simulink model "c00011M_harness"  (R2018a)
settings: Solver=FixedStepAuto  StartTime=0.0  StopTime=300  FixedStep=0.1  RelTol=1e-3
undefined symbols (not defined in the file): A1, hmax, PriorityTank, R1, R2, sigbuilder_block
(part 16 of 73)

== system c00011M_harness/M088/Tank2 ==
  CT2 : Inport
  MR2 : Inport  Port=2
  T2 : Inport  Port=3
  EB2 : Inport  Port=4
  LL1 : Inport  Port=5
  LL3 : Inport  Port=6
  Control : Subsystem
  Logical Operator : Logic  AllPortsSameDT=off  OutDataTypeStr=boolean
  MasterTankControl : Subsystem
  Memory : Memory
  Memory1 : Memory
  Memory2 : Memory
  TankModel : Subsystem
  LL2 : Outport
  wires:
  TankModel/1(LiquidLevel) -> Memory/1, LL2/1
  Control/1(LiquidIn) -> Logical Operator/1
  Control/2(LiquidOut) -> TankModel/2(LiquidOut)
  Memory/1 -> Control/5(LiquidLevel), MasterTankControl/2(LiquidTank2)
  MR2/1 -> Control/3(ManualReference)
  CT2/1 -> Control/2(StartMaintenance), Control/1(ControlType)
  LL3/1 -> Memory2/1
  Memory2/1 -> MasterTankControl/3(LiquidTank3)
  Memory1/1 -> MasterTankControl/1(LiquidTank1)
  EB2/1 -> Control/4(EmergencyButton)
  MasterTankControl/1(AllowTheTankFilling) -> Logical Operator/2
  Logical Operator/1 -> TankModel/1(LiquidIn)
  LL1/1 -> Memory1/1

== system c00011M_harness/M088/Tank3 ==
  CT3 : Inport
  F3 : Inport  Port=2
  E3 : Inport  Port=3
  T3 : Inport  Port=4
  EB3 : Inport  Port=5
  LL1 : Inport  Port=6
  LL2 : Inport  Port=7
  Control : Subsystem
  Logical Operator : Logic  AllPortsSameDT=off  OutDataTypeStr=boolean
  MasterTankControl : Subsystem
  Memory : Memory
  Memory1 : Memory
  Memory2 : Memory
  TankModel : Subsystem
  LL3 : Outport
  wires:
  TankModel/1(LiquidLevel) -> Memory/1, LL3/1
  Control/1(LiquidIn) -> Logical Operator/1
  Control/2(LiquidOut) -> TankModel/2(LiquidOut)
  Memory/1 -> MasterTankControl/3(LiquidTank3), Control/5(LiquidLevel)
  CT3/1 -> Control/1(ControlType)
  F3/1 -> Control/2(Fill)
  E3/1 -> Control/3(Empty)
  LL2/1 -> Memory2/1
  Memory2/1 -> MasterTankControl/2(LiquidTank2)
  Memory1/1 -> MasterTankControl/1(LiquidTank1)
  EB3/1 -> Control/4(EmergencyButton)
  MasterTankControl/1(AllowTheTankFilling) -> Logical Operator/2
  Logical Operator/1 -> TankModel/1(LiquidIn)
  LL1/1 -> Memory1/1

== system c00011M_harness/M089/Tank1 ==
  CT1 : Inport
  MR1 : Inport  Port=2
  T1 : Inport  Port=3
  EB1 : Inport  Port=4
  LL2 : Inport  Port=5
  LL3 : Inport  Port=6
  Control : Subsystem
  Logical Operator : Logic  AllPortsSameDT=off  OutDataTypeStr=boolean
  MasterTankControl : Subsystem
  Memory : Memory
  Memory1 : Memory
  Memory2 : Memory
  TankModel : Subsystem
  LL1 : Outport
  wires:
  TankModel/1(LiquidLevel) -> Memory/1, LL1/1
  Control/1(LiquidIn) -> Logical Operator/1
  Control/2(LiquidOut) -> TankModel/2(LiquidOut)
  Memory/1 -> Control/5(LiquidLevel), MasterTankControl/1(LiquidTank1)
  MR1/1 -> Control/3(ManualReference)
  CT1/1 -> Control/2(StartMaintenance), Control/1(ControlType)
  LL3/1 -> Memory2/1
  Memory2/1 -> MasterTankControl/3(LiquidTank3)
  Memory1/1 -> MasterTankControl/2(LiquidTank2)
  EB1/1 -> Control/4(EmergencyButton)
  MasterTankControl/1(AllowTheTankFilling) -> Logical Operator/2
  Logical Operator/1 -> TankModel/1(LiquidIn)
  LL2/1 -> Memory1/1

== system c00011M_harness/M089/Tank2 ==
  CT2 : Inport
  MR2 : Inport  Port=2
  T2 : Inport  Port=3
  EB2 : Inport  Port=4
  LL1 : Inport  Port=5
  LL3 : Inport  Port=6
  Control : Subsystem
  Logical Operator : Logic  AllPortsSameDT=off  OutDataTypeStr=boolean
  MasterTankControl : Subsystem
  Memory : Memory
  Memory1 : Memory
  Memory2 : Memory
  TankModel : Subsystem
  LL2 : Outport
  wires:
  TankModel/1(LiquidLevel) -> Memory/1, LL2/1
  Control/1(LiquidIn) -> Logical Operator/1
  Control/2(LiquidOut) -> TankModel/2(LiquidOut)
  Memory/1 -> Control/5(LiquidLevel), MasterTankControl/2(LiquidTank2)
  MR2/1 -> Control/3(ManualReference)
  CT2/1 -> Control/2(StartMaintenance), Control/1(ControlType)
  LL3/1 -> Memory2/1
  Memory2/1 -> MasterTankControl/3(LiquidTank3)
  Memory1/1 -> MasterTankControl/1(LiquidTank1)
  EB2/1 -> Control/4(EmergencyButton)
  MasterTankControl/1(AllowTheTankFilling) -> Logical Operator/2
  Logical Operator/1 -> TankModel/1(LiquidIn)
  LL1/1 -> Memory1/1

== system c00011M_harness/M089/Tank3 ==
  CT3 : Inport
  F3 : Inport  Port=2
  E3 : Inport  Port=3
  T3 : Inport  Port=4
  EB3 : Inport  Port=5
  LL1 : Inport  Port=6
  LL2 : Inport  Port=7
  Control : Subsystem
  Logical Operator : Logic  AllPortsSameDT=off  OutDataTypeStr=boolean
  MasterTankControl : Subsystem
  Memory : Memory
  Memory1 : Memory
  Memory2 : Memory
  TankModel : Subsystem
  LL3 : Outport
  wires:
  TankModel/1(LiquidLevel) -> Memory/1, LL3/1
  Control/1(LiquidIn) -> Logical Operator/1
  Control/2(LiquidOut) -> TankModel/2(LiquidOut)
  Memory/1 -> MasterTankControl/3(LiquidTank3), Control/5(LiquidLevel)
  CT3/1 -> Control/1(ControlType)
  F3/1 -> Control/2(Fill)
  E3/1 -> Control/3(Empty)
  LL2/1 -> Memory2/1
  Memory2/1 -> MasterTankControl/2(LiquidTank2)
  Memory1/1 -> MasterTankControl/1(LiquidTank1)
  EB3/1 -> Control/4(EmergencyButton)
  MasterTankControl/1(AllowTheTankFilling) -> Logical Operator/2
  Logical Operator/1 -> TankModel/1(LiquidIn)
  LL1/1 -> Memory1/1

== system c00011M_harness/M090/Tank1 ==
  CT1 : Inport
  MR1 : Inport  Port=2
  T1 : Inport  Port=3
  EB1 : Inport  Port=4
  LL2 : Inport  Port=5
  LL3 : Inport  Port=6
  Control : Subsystem
  Logical Operator : Logic  AllPortsSameDT=off  OutDataTypeStr=boolean
  MasterTankControl : Subsystem
  Memory : Memory
  Memory1 : Memory
  Memory2 : Memory
  TankModel : Subsystem
  LL1 : Outport
  wires:
  TankModel/1(LiquidLevel) -> Memory/1, LL1/1
  Control/1(LiquidIn) -> Logical Operator/1
  Control/2(LiquidOut) -> TankModel/2(LiquidOut)
  Memory/1 -> Control/5(LiquidLevel), MasterTankControl/1(LiquidTank1)
  MR1/1 -> Control/3(ManualReference)
  CT1/1 -> Control/2(StartMaintenance), Control/1(ControlType)
  LL3/1 -> Memory2/1
  Memory2/1 -> MasterTankControl/3(LiquidTank3)
  Memory1/1 -> MasterTankControl/2(LiquidTank2)
  EB1/1 -> Control/4(EmergencyButton)
  MasterTankControl/1(AllowTheTankFilling) -> Logical Operator/2
  Logical Operator/1 -> TankModel/1(LiquidIn)
  LL2/1 -> Memory1/1

== system c00011M_harness/M090/Tank2 ==
  CT2 : Inport
  MR2 : Inport  Port=2
  T2 : Inport  Port=3
  EB2 : Inport  Port=4
  LL1 : Inport  Port=5
  LL3 : Inport  Port=6
  Control : Subsystem
  Logical Operator : Logic  AllPortsSameDT=off  OutDataTypeStr=boolean
  MasterTankControl : Subsystem
  Memory : Memory
  Memory1 : Memory
  Memory2 : Memory
  TankModel : Subsystem
  LL2 : Outport
  wires:
  TankModel/1(LiquidLevel) -> Memory/1, LL2/1
  Control/1(LiquidIn) -> Logical Operator/1
  Control/2(LiquidOut) -> TankModel/2(LiquidOut)
  Memory/1 -> Control/5(LiquidLevel), MasterTankControl/2(LiquidTank2)
  MR2/1 -> Control/3(ManualReference)
  CT2/1 -> Control/2(StartMaintenance), Control/1(ControlType)
  LL3/1 -> Memory2/1
  Memory2/1 -> MasterTankControl/3(LiquidTank3)
  Memory1/1 -> MasterTankControl/1(LiquidTank1)
  EB2/1 -> Control/4(EmergencyButton)
  MasterTankControl/1(AllowTheTankFilling) -> Logical Operator/2
  Logical Operator/1 -> TankModel/1(LiquidIn)
  LL1/1 -> Memory1/1

== system c00011M_harness/M090/Tank3 ==
  CT3 : Inport
  F3 : Inport  Port=2
  E3 : Inport  Port=3
  T3 : Inport  Port=4
  EB3 : Inport  Port=5
  LL1 : Inport  Port=6
  LL2 : Inport  Port=7
  Control : Subsystem
  Logical Operator : Logic  AllPortsSameDT=off  OutDataTypeStr=boolean
  MasterTankControl : Subsystem
  Memory : Memory
  Memory1 : Memory
  Memory2 : Memory
  TankModel : Subsystem
  LL3 : Outport
  wires:
  TankModel/1(LiquidLevel) -> Memory/1, LL3/1
  Control/1(LiquidIn) -> Logical Operator/1
  Control/2(LiquidOut) -> TankModel/2(LiquidOut)
  Memory/1 -> MasterTankControl/3(LiquidTank3), Control/5(LiquidLevel)
  CT3/1 -> Control/1(ControlType)
  F3/1 -> Control/2(Fill)
  E3/1 -> Control/3(Empty)
  LL2/1 -> Memory2/1
  Memory2/1 -> MasterTankControl/2(LiquidTank2)
  Memory1/1 -> MasterTankControl/1(LiquidTank1)
  EB3/1 -> Control/4(EmergencyButton)
  MasterTankControl/1(AllowTheTankFilling) -> Logical Operator/2
  Logical Operator/1 -> TankModel/1(LiquidIn)
  LL1/1 -> Memory1/1

== system c00011M_harness/M091/Tank1 ==
  CT1 : Inport
  MR1 : Inport  Port=2
  T1 : Inport  Port=3
  EB1 : Inport  Port=4
  LL2 : Inport  Port=5
  LL3 : Inport  Port=6
  Control : Subsystem
  Logical Operator : Logic  AllPortsSameDT=off  OutDataTypeStr=boolean
  MasterTankControl : Subsystem
  Memory : Memory
  Memory1 : Memory
  Memory2 : Memory
  TankModel : Subsystem
  LL1 : Outport
  wires:
  TankModel/1(LiquidLevel) -> Memory/1, LL1/1
  Control/1(LiquidIn) -> Logical Operator/1
  Control/2(LiquidOut) -> TankModel/2(LiquidOut)
  Memory/1 -> Control/5(LiquidLevel), MasterTankControl/1(LiquidTank1)
  MR1/1 -> Control/3(ManualReference)
  CT1/1 -> Control/2(StartMaintenance), Control/1(ControlType)
  LL3/1 -> Memory2/1
  Memory2/1 -> MasterTankControl/3(LiquidTank3)
  Memory1/1 -> MasterTankControl/2(LiquidTank2)
  EB1/1 -> Control/4(EmergencyButton)
  MasterTankControl/1(AllowTheTankFilling) -> Logical Operator/2
  Logical Operator/1 -> TankModel/1(LiquidIn)
  LL2/1 -> Memory1/1

== system c00011M_harness/M091/Tank2 ==
  CT2 : Inport
  MR2 : Inport  Port=2
  T2 : Inport  Port=3
  EB2 : Inport  Port=4
  LL1 : Inport  Port=5
  LL3 : Inport  Port=6
  Control : Subsystem
  Logical Operator : Logic  AllPortsSameDT=off  OutDataTypeStr=boolean
  MasterTankControl : Subsystem
  Memory : Memory
  Memory1 : Memory
  Memory2 : Memory
  TankModel : Subsystem
  LL2 : Outport
  wires:
  TankModel/1(LiquidLevel) -> Memory/1, LL2/1
  Control/1(LiquidIn) -> Logical Operator/1
  Control/2(LiquidOut) -> TankModel/2(LiquidOut)
  Memory/1 -> Control/5(LiquidLevel), MasterTankControl/2(LiquidTank2)
  MR2/1 -> Control/3(ManualReference)
  CT2/1 -> Control/2(StartMaintenance), Control/1(ControlType)
  LL3/1 -> Memory2/1
  Memory2/1 -> MasterTankControl/3(LiquidTank3)
  Memory1/1 -> MasterTankControl/1(LiquidTank1)
  EB2/1 -> Control/4(EmergencyButton)
  MasterTankControl/1(AllowTheTankFilling) -> Logical Operator/2
  Logical Operator/1 -> TankModel/1(LiquidIn)
  LL1/1 -> Memory1/1

== system c00011M_harness/M091/Tank3 ==
  CT3 : Inport
  F3 : Inport  Port=2
  E3 : Inport  Port=3
  T3 : Inport  Port=4
  EB3 : Inport  Port=5
  LL1 : Inport  Port=6
  LL2 : Inport  Port=7
  Control : Subsystem
  Logical Operator : Logic  AllPortsSameDT=off  OutDataTypeStr=boolean
  MasterTankControl : Subsystem
  Memory : Memory
  Memory1 : Memory
  Memory2 : Memory
  TankModel : Subsystem
  LL3 : Outport
  wires:
  TankModel/1(LiquidLevel) -> Memory/1, LL3/1
  Control/1(LiquidIn) -> Logical Operator/1
  Control/2(LiquidOut) -> TankModel/2(LiquidOut)
  Memory/1 -> MasterTankControl/3(LiquidTank3), Control/5(LiquidLevel)
  CT3/1 -> Control/1(ControlType)
  F3/1 -> Control/2(Fill)
  E3/1 -> Control/3(Empty)
  LL2/1 -> Memory2/1
  Memory2/1 -> MasterTankControl/2(LiquidTank2)
  Memory1/1 -> MasterTankControl/1(LiquidTank1)
  EB3/1 -> Control/4(EmergencyButton)
  MasterTankControl/1(AllowTheTankFilling) -> Logical Operator/2
  Logical Operator/1 -> TankModel/1(LiquidIn)
  LL1/1 -> Memory1/1

== system c00011M_harness/M092/Tank1 ==
  CT1 : Inport
  MR1 : Inport  Port=2
  T1 : Inport  Port=3
  EB1 : Inport  Port=4
  LL2 : Inport  Port=5
  LL3 : Inport  Port=6
  Control : Subsystem
  Logical Operator : Logic  AllPortsSameDT=off  OutDataTypeStr=boolean
  MasterTankControl : Subsystem
  Memory : Memory
  Memory1 : Memory
  Memory2 : Memory
  TankModel : Subsystem
  LL1 : Outport
  wires:
  TankModel/1(LiquidLevel) -> Memory/1, LL1/1
  Control/1(LiquidIn) -> Logical Operator/1
  Control/2(LiquidOut) -> TankModel/2(LiquidOut)
  Memory/1 -> Control/5(LiquidLevel), MasterTankControl/1(LiquidTank1)
  MR1/1 -> Control/3(ManualReference)
  CT1/1 -> Control/2(StartMaintenance), Control/1(ControlType)
  LL3/1 -> Memory2/1
  Memory2/1 -> MasterTankControl/3(LiquidTank3)
  Memory1/1 -> MasterTankControl/2(LiquidTank2)
  EB1/1 -> Control/4(EmergencyButton)
  MasterTankControl/1(AllowTheTankFilling) -> Logical Operator/2
  Logical Operator/1 -> TankModel/1(LiquidIn)
  LL2/1 -> Memory1/1

== system c00011M_harness/M092/Tank2 ==
  CT2 : Inport
  MR2 : Inport  Port=2
  T2 : Inport  Port=3
  EB2 : Inport  Port=4
  LL1 : Inport  Port=5
  LL3 : Inport  Port=6
  Control : Subsystem
  Logical Operator : Logic  AllPortsSameDT=off  OutDataTypeStr=boolean
  MasterTankControl : Subsystem
  Memory : Memory
  Memory1 : Memory
  Memory2 : Memory
  TankModel : Subsystem
  LL2 : Outport
  wires:
  TankModel/1(LiquidLevel) -> Memory/1, LL2/1
  Control/1(LiquidIn) -> Logical Operator/1
  Control/2(LiquidOut) -> TankModel/2(LiquidOut)
  Memory/1 -> Control/5(LiquidLevel), MasterTankControl/2(LiquidTank2)
  MR2/1 -> Control/3(ManualReference)
  CT2/1 -> Control/2(StartMaintenance), Control/1(ControlType)
  LL3/1 -> Memory2/1
  Memory2/1 -> MasterTankControl/3(LiquidTank3)
  Memory1/1 -> MasterTankControl/1(LiquidTank1)
  EB2/1 -> Control/4(EmergencyButton)
  MasterTankControl/1(AllowTheTankFilling) -> Logical Operator/2
  Logical Operator/1 -> TankModel/1(LiquidIn)
  LL1/1 -> Memory1/1

== system c00011M_harness/M092/Tank3 ==
  CT3 : Inport
  F3 : Inport  Port=2
  E3 : Inport  Port=3
  T3 : Inport  Port=4
  EB3 : Inport  Port=5
  LL1 : Inport  Port=6
  LL2 : Inport  Port=7
  Control : Subsystem
  Logical Operator : Logic  AllPortsSameDT=off  OutDataTypeStr=boolean
  MasterTankControl : Subsystem
  Memory : Memory
  Memory1 : Memory
  Memory2 : Memory
  TankModel : Subsystem
  LL3 : Outport
  wires:
  TankModel/1(LiquidLevel) -> Memory/1, LL3/1
  Control/1(LiquidIn) -> Logical Operator/1
  Control/2(LiquidOut) -> TankModel/2(LiquidOut)
  Memory/1 -> MasterTankControl/3(LiquidTank3), Control/5(LiquidLevel)
  CT3/1 -> Control/1(ControlType)
  F3/1 -> Control/2(Fill)
  E3/1 -> Control/3(Empty)
  LL2/1 -> Memory2/1
  Memory2/1 -> MasterTankControl/2(LiquidTank2)
  Memory1/1 -> MasterTankControl/1(LiquidTank1)
  EB3/1 -> Control/4(EmergencyButton)
  MasterTankControl/1(AllowTheTankFilling) -> Logical Operator/2
  Logical Operator/1 -> TankModel/1(LiquidIn)
  LL1/1 -> Memory1/1

== system c00011M_harness/M093/Tank1 ==
  CT1 : Inport
  MR1 : Inport  Port=2
  T1 : Inport  Port=3
  EB1 : Inport  Port=4
  LL2 : Inport  Port=5
  LL3 : Inport  Port=6
  Control : Subsystem
  Logical Operator : Logic  AllPortsSameDT=off  OutDataTypeStr=boolean
  MasterTankControl : Subsystem
  Memory : Memory
  Memory1 : Memory
  Memory2 : Memory
  TankModel : Subsystem
  LL1 : Outport
  wires:
  TankModel/1(LiquidLevel) -> Memory/1, LL1/1
  Control/1(LiquidIn) -> Logical Operator/1
  Control/2(LiquidOut) -> TankModel/2(LiquidOut)
  Memory/1 -> Control/5(LiquidLevel), MasterTankControl/1(LiquidTank1)
  MR1/1 -> Control/3(ManualReference)
  CT1/1 -> Control/2(StartMaintenance), Control/1(ControlType)
  LL3/1 -> Memory2/1
  Memory2/1 -> MasterTankControl/3(LiquidTank3)
  Memory1/1 -> MasterTankControl/2(LiquidTank2)
  EB1/1 -> Control/4(EmergencyButton)
  MasterTankControl/1(AllowTheTankFilling) -> Logical Operator/2
  Logical Operator/1 -> TankModel/1(LiquidIn)
  LL2/1 -> Memory1/1

== system c00011M_harness/M093/Tank2 ==
  CT2 : Inport
  MR2 : Inport  Port=2
  T2 : Inport  Port=3
  EB2 : Inport  Port=4
  LL1 : Inport  Port=5
  LL3 : Inport  Port=6
  Control : Subsystem
  Logical Operator : Logic  AllPortsSameDT=off  OutDataTypeStr=boolean
  MasterTankControl : Subsystem
  Memory : Memory
  Memory1 : Memory
  Memory2 : Memory
  TankModel : Subsystem
  LL2 : Outport
  wires:
  TankModel/1(LiquidLevel) -> Memory/1, LL2/1
  Control/1(LiquidIn) -> Logical Operator/1
  Control/2(LiquidOut) -> TankModel/2(LiquidOut)
  Memory/1 -> Control/5(LiquidLevel), MasterTankControl/2(LiquidTank2)
  MR2/1 -> Control/3(ManualReference)
  CT2/1 -> Control/2(StartMaintenance), Control/1(ControlType)
  LL3/1 -> Memory2/1
  Memory2/1 -> MasterTankControl/3(LiquidTank3)
  Memory1/1 -> MasterTankControl/1(LiquidTank1)
  EB2/1 -> Control/4(EmergencyButton)
  MasterTankControl/1(AllowTheTankFilling) -> Logical Operator/2
  Logical Operator/1 -> TankModel/1(LiquidIn)
  LL1/1 -> Memory1/1

== system c00011M_harness/M093/Tank3 ==
  CT3 : Inport
  F3 : Inport  Port=2
  E3 : Inport  Port=3
  T3 : Inport  Port=4
  EB3 : Inport  Port=5
  LL1 : Inport  Port=6
  LL2 : Inport  Port=7
  Control : Subsystem
  Logical Operator : Logic  AllPortsSameDT=off  OutDataTypeStr=boolean
  MasterTankControl : Subsystem
  Memory : Memory
  Memory1 : Memory
  Memory2 : Memory
  TankModel : Subsystem
  LL3 : Outport
  wires:
  TankModel/1(LiquidLevel) -> Memory/1, LL3/1
  Control/1(LiquidIn) -> Logical Operator/1
  Control/2(LiquidOut) -> TankModel/2(LiquidOut)
  Memory/1 -> MasterTankControl/3(LiquidTank3), Control/5(LiquidLevel)
  CT3/1 -> Control/1(ControlType)
  F3/1 -> Control/2(Fill)
  E3/1 -> Control/3(Empty)
  LL2/1 -> Memory2/1
  Memory2/1 -> MasterTankControl/2(LiquidTank2)
  Memory1/1 -> MasterTankControl/1(LiquidTank1)
  EB3/1 -> Control/4(EmergencyButton)
  MasterTankControl/1(AllowTheTankFilling) -> Logical Operator/2
  Logical Operator/1 -> TankModel/1(LiquidIn)
  LL1/1 -> Memory1/1

== system c00011M_harness/M094/Tank1 ==
  CT1 : Inport
  MR1 : Inport  Port=2
  T1 : Inport  Port=3
  EB1 : Inport  Port=4
  LL2 : Inport  Port=5
  LL3 : Inport  Port=6
  Control : Subsystem
  Logical Operator : Logic  AllPortsSameDT=off  OutDataTypeStr=boolean
  MasterTankControl : Subsystem
  Memory : Memory
  Memory1 : Memory
  Memory2 : Memory
  TankModel : Subsystem
  LL1 : Outport
  wires:
  TankModel/1(LiquidLevel) -> Memory/1, LL1/1
  Control/1(LiquidIn) -> Logical Operator/1
  Control/2(LiquidOut) -> TankModel/2(LiquidOut)
  Memory/1 -> Control/5(LiquidLevel), MasterTankControl/1(LiquidTank1)
  MR1/1 -> Control/3(ManualReference)
  CT1/1 -> Control/2(StartMaintenance), Control/1(ControlType)
  LL3/1 -> Memory2/1
  Memory2/1 -> MasterTankControl/3(LiquidTank3)
  Memory1/1 -> MasterTankControl/2(LiquidTank2)
  EB1/1 -> Control/4(EmergencyButton)
  MasterTankControl/1(AllowTheTankFilling) -> Logical Operator/2
  Logical Operator/1 -> TankModel/1(LiquidIn)
  LL2/1 -> Memory1/1

== system c00011M_harness/M094/Tank2 ==
  CT2 : Inport
  MR2 : Inport  Port=2
  T2 : Inport  Port=3
  EB2 : Inport  Port=4
  LL1 : Inport  Port=5
  LL3 : Inport  Port=6
  Control : Subsystem
  Logical Operator : Logic  AllPortsSameDT=off  OutDataTypeStr=boolean
  MasterTankControl : Subsystem
  Memory : Memory
  Memory1 : Memory
  Memory2 : Memory
  TankModel : Subsystem
  LL2 : Outport
  wires:
  TankModel/1(LiquidLevel) -> Memory/1, LL2/1
  Control/1(LiquidIn) -> Logical Operator/1
  Control/2(LiquidOut) -> TankModel/2(LiquidOut)
  Memory/1 -> Control/5(LiquidLevel), MasterTankControl/2(LiquidTank2)
  MR2/1 -> Control/3(ManualReference)
  CT2/1 -> Control/2(StartMaintenance), Control/1(ControlType)
  LL3/1 -> Memory2/1
  Memory2/1 -> MasterTankControl/3(LiquidTank3)
  Memory1/1 -> MasterTankControl/1(LiquidTank1)
  EB2/1 -> Control/4(EmergencyButton)
  MasterTankControl/1(AllowTheTankFilling) -> Logical Operator/2
  Logical Operator/1 -> TankModel/1(LiquidIn)
  LL1/1 -> Memory1/1

== system c00011M_harness/M094/Tank3 ==
  CT3 : Inport
  F3 : Inport  Port=2
  E3 : Inport  Port=3
  T3 : Inport  Port=4
  EB3 : Inport  Port=5
  LL1 : Inport  Port=6
  LL2 : Inport  Port=7
  Control : Subsystem
  Logical Operator : Logic  AllPortsSameDT=off  OutDataTypeStr=boolean
  MasterTankControl : Subsystem
  Memory : Memory
  Memory1 : Memory
  Memory2 : Memory
  TankModel : Subsystem
  LL3 : Outport
  wires:
  TankModel/1(LiquidLevel) -> Memory/1, LL3/1
  Control/1(LiquidIn) -> Logical Operator/1
  Control/2(LiquidOut) -> TankModel/2(LiquidOut)
  Memory/1 -> MasterTankControl/3(LiquidTank3), Control/5(LiquidLevel)
  CT3/1 -> Control/1(ControlType)
  F3/1 -> Control/2(Fill)
  E3/1 -> Control/3(Empty)
  LL2/1 -> Memory2/1
  Memory2/1 -> MasterTankControl/2(LiquidTank2)
  Memory1/1 -> MasterTankControl/1(LiquidTank1)
  EB3/1 -> Control/4(EmergencyButton)
  MasterTankControl/1(AllowTheTankFilling) -> Logical Operator/2
  Logical Operator/1 -> TankModel/1(LiquidIn)
  LL1/1 -> Memory1/1

== system c00011M_harness/M095/Tank1 ==
  CT1 : Inport
  MR1 : Inport  Port=2
  T1 : Inport  Port=3
  EB1 : Inport  Port=4
  LL2 : Inport  Port=5
  LL3 : Inport  Port=6
  Control : Subsystem
  Logical Operator : Logic  AllPortsSameDT=off  OutDataTypeStr=boolean
  MasterTankControl : Subsystem
  Memory : Memory
  Memory1 : Memory
  Memory2 : Memory
  TankModel : Subsystem
  LL1 : Outport
  wires:
  TankModel/1(LiquidLevel) -> Memory/1, LL1/1
  Control/1(LiquidIn) -> Logical Operator/1
  Control/2(LiquidOut) -> TankModel/2(LiquidOut)
  Memory/1 -> Control/5(LiquidLevel), MasterTankControl/1(LiquidTank1)
  MR1/1 -> Control/3(ManualReference)
  CT1/1 -> Control/2(StartMaintenance), Control/1(ControlType)
  LL3/1 -> Memory2/1
  Memory2/1 -> MasterTankControl/3(LiquidTank3)
  Memory1/1 -> MasterTankControl/2(LiquidTank2)
  EB1/1 -> Control/4(EmergencyButton)
  MasterTankControl/1(AllowTheTankFilling) -> Logical Operator/2
  Logical Operator/1 -> TankModel/1(LiquidIn)
  LL2/1 -> Memory1/1

== system c00011M_harness/M095/Tank2 ==
  CT2 : Inport
  MR2 : Inport  Port=2
  T2 : Inport  Port=3
  EB2 : Inport  Port=4
  LL1 : Inport  Port=5
  LL3 : Inport  Port=6
  Control : Subsystem
  Logical Operator : Logic  AllPortsSameDT=off  OutDataTypeStr=boolean
  MasterTankControl : Subsystem
  Memory : Memory
  Memory1 : Memory
  Memory2 : Memory
  TankModel : Subsystem
  LL2 : Outport
  wires:
  TankModel/1(LiquidLevel) -> Memory/1, LL2/1
  Control/1(LiquidIn) -> Logical Operator/1
  Control/2(LiquidOut) -> TankModel/2(LiquidOut)
  Memory/1 -> Control/5(LiquidLevel), MasterTankControl/2(LiquidTank2)
  MR2/1 -> Control/3(ManualReference)
  CT2/1 -> Control/2(StartMaintenance), Control/1(ControlType)
  LL3/1 -> Memory2/1
  Memory2/1 -> MasterTankControl/3(LiquidTank3)
  Memory1/1 -> MasterTankControl/1(LiquidTank1)
  EB2/1 -> Control/4(EmergencyButton)
  MasterTankControl/1(AllowTheTankFilling) -> Logical Operator/2
  Logical Operator/1 -> TankModel/1(LiquidIn)
  LL1/1 -> Memory1/1

== system c00011M_harness/M095/Tank3 ==
  CT3 : Inport
  F3 : Inport  Port=2
  E3 : Inport  Port=3
  T3 : Inport  Port=4
  EB3 : Inport  Port=5
  LL1 : Inport  Port=6
  LL2 : Inport  Port=7
  Control : Subsystem
  Logical Operator : Logic  AllPortsSameDT=off  OutDataTypeStr=boolean
  MasterTankControl : Subsystem
  Memory : Memory
  Memory1 : Memory
  Memory2 : Memory
  TankModel : Subsystem
  LL3 : Outport
  wires:
  TankModel/1(LiquidLevel) -> Memory/1, LL3/1
  Control/1(LiquidIn) -> Logical Operator/1
  Control/2(LiquidOut) -> TankModel/2(LiquidOut)
  Memory/1 -> MasterTankControl/3(LiquidTank3), Control/5(LiquidLevel)
  CT3/1 -> Control/1(ControlType)
  F3/1 -> Control/2(Fill)
  E3/1 -> Control/3(Empty)
  LL2/1 -> Memory2/1
  Memory2/1 -> MasterTankControl/2(LiquidTank2)
  Memory1/1 -> MasterTankControl/1(LiquidTank1)
  EB3/1 -> Control/4(EmergencyButton)
  MasterTankControl/1(AllowTheTankFilling) -> Logical Operator/2
  Logical Operator/1 -> TankModel/1(LiquidIn)
  LL1/1 -> Memory1/1

== system c00011M_harness/M096/Tank1 ==
  CT1 : Inport
  MR1 : Inport  Port=2
  T1 : Inport  Port=3
  EB1 : Inport  Port=4
  LL2 : Inport  Port=5
  LL3 : Inport  Port=6
  Control : Subsystem
  Logical Operator : Logic  AllPortsSameDT=off  OutDataTypeStr=boolean
  MasterTankControl : Subsystem
  Memory : Memory
  Memory1 : Memory
  Memory2 : Memory
  TankModel : Subsystem
  LL1 : Outport
  wires:
  TankModel/1(LiquidLevel) -> Memory/1, LL1/1
  Control/1(LiquidIn) -> Logical Operator/1
  Control/2(LiquidOut) -> TankModel/2(LiquidOut)
  Memory/1 -> Control/5(LiquidLevel), MasterTankControl/1(LiquidTank1)
  MR1/1 -> Control/3(ManualReference)
  CT1/1 -> Control/2(StartMaintenance), Control/1(ControlType)
  LL3/1 -> Memory2/1
  Memory2/1 -> MasterTankControl/3(LiquidTank3)
  Memory1/1 -> MasterTankControl/2(LiquidTank2)
  EB1/1 -> Control/4(EmergencyButton)
  MasterTankControl/1(AllowTheTankFilling) -> Logical Operator/2
  Logical Operator/1 -> TankModel/1(LiquidIn)
  LL2/1 -> Memory1/1

== system c00011M_harness/M096/Tank2 ==
  CT2 : Inport
  MR2 : Inport  Port=2
  T2 : Inport  Port=3
  EB2 : Inport  Port=4
  LL1 : Inport  Port=5
  LL3 : Inport  Port=6
  Control : Subsystem
  Logical Operator : Logic  AllPortsSameDT=off  OutDataTypeStr=boolean
  MasterTankControl : Subsystem
  Memory : Memory
  Memory1 : Memory
  Memory2 : Memory
  TankModel : Subsystem
  LL2 : Outport
  wires:
  TankModel/1(LiquidLevel) -> Memory/1, LL2/1
  Control/1(LiquidIn) -> Logical Operator/1
  Control/2(LiquidOut) -> TankModel/2(LiquidOut)
  Memory/1 -> Control/5(LiquidLevel), MasterTankControl/2(LiquidTank2)
  MR2/1 -> Control/3(ManualReference)
  CT2/1 -> Control/2(StartMaintenance), Control/1(ControlType)
  LL3/1 -> Memory2/1
  Memory2/1 -> MasterTankControl/3(LiquidTank3)
  Memory1/1 -> MasterTankControl/1(LiquidTank1)
  EB2/1 -> Control/4(EmergencyButton)
  MasterTankControl/1(AllowTheTankFilling) -> Logical Operator/2
  Logical Operator/1 -> TankModel/1(LiquidIn)
  LL1/1 -> Memory1/1

== system c00011M_harness/M096/Tank3 ==
  CT3 : Inport
  F3 : Inport  Port=2
  E3 : Inport  Port=3
  T3 : Inport  Port=4
  EB3 : Inport  Port=5
  LL1 : Inport  Port=6
  LL2 : Inport  Port=7
  Control : Subsystem
  Logical Operator : Logic  AllPortsSameDT=off  OutDataTypeStr=boolean
  MasterTankControl : Subsystem
  Memory : Memory
  Memory1 : Memory
  Memory2 : Memory
  TankModel : Subsystem
  LL3 : Outport
  wires:
  TankModel/1(LiquidLevel) -> Memory/1, LL3/1
  Control/1(LiquidIn) -> Logical Operator/1
  Control/2(LiquidOut) -> TankModel/2(LiquidOut)
  Memory/1 -> MasterTankControl/3(LiquidTank3), Control/5(LiquidLevel)
  CT3/1 -> Control/1(ControlType)
  F3/1 -> Control/2(Fill)
  E3/1 -> Control/3(Empty)
  LL2/1 -> Memory2/1
  Memory2/1 -> MasterTankControl/2(LiquidTank2)
  Memory1/1 -> MasterTankControl/1(LiquidTank1)
  EB3/1 -> Control/4(EmergencyButton)
  MasterTankControl/1(AllowTheTankFilling) -> Logical Operator/2
  Logical Operator/1 -> TankModel/1(LiquidIn)
  LL1/1 -> Memory1/1

== system c00011M_harness/M097/Tank1 ==
  CT1 : Inport
  MR1 : Inport  Port=2
  T1 : Inport  Port=3
  EB1 : Inport  Port=4
  LL2 : Inport  Port=5
  LL3 : Inport  Port=6
  Control : Subsystem
  Logical Operator : Logic  AllPortsSameDT=off  OutDataTypeStr=boolean
  MasterTankControl : Subsystem
  Memory : Memory
  Memory1 : Memory
  Memory2 : Memory
  TankModel : Subsystem
  LL1 : Outport
  wires:
  TankModel/1(LiquidLevel) -> Memory/1, LL1/1
  Control/1(LiquidIn) -> Logical Operator/1
  Control/2(LiquidOut) -> TankModel/2(LiquidOut)
  Memory/1 -> Control/5(LiquidLevel), MasterTankControl/1(LiquidTank1)
  MR1/1 -> Control/3(ManualReference)
  CT1/1 -> Control/2(StartMaintenance), Control/1(ControlType)
  LL3/1 -> Memory2/1
  Memory2/1 -> MasterTankControl/3(LiquidTank3)
  Memory1/1 -> MasterTankControl/2(LiquidTank2)
  EB1/1 -> Control/4(EmergencyButton)
  MasterTankControl/1(AllowTheTankFilling) -> Logical Operator/2
  Logical Operator/1 -> TankModel/1(LiquidIn)
  LL2/1 -> Memory1/1

== system c00011M_harness/M097/Tank2 ==
  CT2 : Inport
  MR2 : Inport  Port=2
  T2 : Inport  Port=3
  EB2 : Inport  Port=4
  LL1 : Inport  Port=5
  LL3 : Inport  Port=6
  Control : Subsystem
  Logical Operator : Logic  AllPortsSameDT=off  OutDataTypeStr=boolean
  MasterTankControl : Subsystem
  Memory : Memory
  Memory1 : Memory
  Memory2 : Memory
  TankModel : Subsystem
  LL2 : Outport
  wires:
  TankModel/1(LiquidLevel) -> Memory/1, LL2/1
  Control/1(LiquidIn) -> Logical Operator/1
  Control/2(LiquidOut) -> TankModel/2(LiquidOut)
  Memory/1 -> Control/5(LiquidLevel), MasterTankControl/2(LiquidTank2)
  MR2/1 -> Control/3(ManualReference)
  CT2/1 -> Control/2(StartMaintenance), Control/1(ControlType)
  LL3/1 -> Memory2/1
  Memory2/1 -> MasterTankControl/3(LiquidTank3)
  Memory1/1 -> MasterTankControl/1(LiquidTank1)
  EB2/1 -> Control/4(EmergencyButton)
  MasterTankControl/1(AllowTheTankFilling) -> Logical Operator/2
  Logical Operator/1 -> TankModel/1(LiquidIn)
  LL1/1 -> Memory1/1

== system c00011M_harness/M097/Tank3 ==
  CT3 : Inport
  F3 : Inport  Port=2
  E3 : Inport  Port=3
  T3 : Inport  Port=4
  EB3 : Inport  Port=5
  LL1 : Inport  Port=6
  LL2 : Inport  Port=7
  Control : Subsystem
  Logical Operator : Logic  AllPortsSameDT=off  OutDataTypeStr=boolean
  MasterTankControl : Subsystem
  Memory : Memory
  Memory1 : Memory
  Memory2 : Memory
  TankModel : Subsystem
  LL3 : Outport
  wires:
  TankModel/1(LiquidLevel) -> Memory/1, LL3/1
  Control/1(LiquidIn) -> Logical Operator/1
  Control/2(LiquidOut) -> TankModel/2(LiquidOut)
  Memory/1 -> MasterTankControl/3(LiquidTank3), Control/5(LiquidLevel)
  CT3/1 -> Control/1(ControlType)
  F3/1 -> Control/2(Fill)
  E3/1 -> Control/3(Empty)
  LL2/1 -> Memory2/1
  Memory2/1 -> MasterTankControl/2(LiquidTank2)
  Memory1/1 -> MasterTankControl/1(LiquidTank1)
  EB3/1 -> Control/4(EmergencyButton)
  MasterTankControl/1(AllowTheTankFilling) -> Logical Operator/2
  Logical Operator/1 -> TankModel/1(LiquidIn)
  LL1/1 -> Memory1/1

== system c00011M_harness/M098/Tank1 ==
  CT1 : Inport
  MR1 : Inport  Port=2
  T1 : Inport  Port=3
  EB1 : Inport  Port=4
  LL2 : Inport  Port=5
  LL3 : Inport  Port=6
  Control : Subsystem
  Logical Operator : Logic  AllPortsSameDT=off  OutDataTypeStr=boolean
  MasterTankControl : Subsystem
  Memory : Memory
  Memory1 : Memory
  Memory2 : Memory
  TankModel : Subsystem
  LL1 : Outport
  wires:
  TankModel/1(LiquidLevel) -> Memory/1, LL1/1
  Control/1(LiquidIn) -> Logical Operator/1
  Control/2(LiquidOut) -> TankModel/2(LiquidOut)
  Memory/1 -> Control/5(LiquidLevel), MasterTankControl/1(LiquidTank1)
  MR1/1 -> Control/3(ManualReference)
  CT1/1 -> Control/2(StartMaintenance), Control/1(ControlType)
  LL3/1 -> Memory2/1
  Memory2/1 -> MasterTankControl/3(LiquidTank3)
  Memory1/1 -> MasterTankControl/2(LiquidTank2)
  EB1/1 -> Control/4(EmergencyButton)
  MasterTankControl/1(AllowTheTankFilling) -> Logical Operator/2
  Logical Operator/1 -> TankModel/1(LiquidIn)
  LL2/1 -> Memory1/1

== system c00011M_harness/M098/Tank2 ==
  CT2 : Inport
  MR2 : Inport  Port=2
  T2 : Inport  Port=3
  EB2 : Inport  Port=4
  LL1 : Inport  Port=5
  LL3 : Inport  Port=6
  Control : Subsystem
  Logical Operator : Logic  AllPortsSameDT=off  OutDataTypeStr=boolean
  MasterTankControl : Subsystem
  Memory : Memory
  Memory1 : Memory
  Memory2 : Memory
  TankModel : Subsystem
  LL2 : Outport
  wires:
  TankModel/1(LiquidLevel) -> Memory/1, LL2/1
  Control/1(LiquidIn) -> Logical Operator/1
  Control/2(LiquidOut) -> TankModel/2(LiquidOut)
  Memory/1 -> Control/5(LiquidLevel), MasterTankControl/2(LiquidTank2)
  MR2/1 -> Control/3(ManualReference)
  CT2/1 -> Control/2(StartMaintenance), Control/1(ControlType)
  LL3/1 -> Memory2/1
  Memory2/1 -> MasterTankControl/3(LiquidTank3)
  Memory1/1 -> MasterTankControl/1(LiquidTank1)
  EB2/1 -> Control/4(EmergencyButton)
  MasterTankControl/1(AllowTheTankFilling) -> Logical Operator/2
  Logical Operator/1 -> TankModel/1(LiquidIn)
  LL1/1 -> Memory1/1

== system c00011M_harness/M098/Tank3 ==
  CT3 : Inport
  F3 : Inport  Port=2
  E3 : Inport  Port=3
  T3 : Inport  Port=4
  EB3 : Inport  Port=5
  LL1 : Inport  Port=6
  LL2 : Inport  Port=7
  Control : Subsystem
  Logical Operator : Logic  AllPortsSameDT=off  OutDataTypeStr=boolean
  MasterTankControl : Subsystem
  Memory : Memory
  Memory1 : Memory
  Memory2 : Memory
  TankModel : Subsystem
  LL3 : Outport
  wires:
  TankModel/1(LiquidLevel) -> Memory/1, LL3/1
  Control/1(LiquidIn) -> Logical Operator/1
  Control/2(LiquidOut) -> TankModel/2(LiquidOut)
  Memory/1 -> MasterTankControl/3(LiquidTank3), Control/5(LiquidLevel)
  CT3/1 -> Control/1(ControlType)
  F3/1 -> Control/2(Fill)
  E3/1 -> Control/3(Empty)
  LL2/1 -> Memory2/1
  Memory2/1 -> MasterTankControl/2(LiquidTank2)
  Memory1/1 -> MasterTankControl/1(LiquidTank1)
  EB3/1 -> Control/4(EmergencyButton)
  MasterTankControl/1(AllowTheTankFilling) -> Logical Operator/2
  Logical Operator/1 -> TankModel/1(LiquidIn)
  LL1/1 -> Memory1/1

== system c00011M_harness/M099/Tank1 ==
  CT1 : Inport
  MR1 : Inport  Port=2
  T1 : Inport  Port=3
  EB1 : Inport  Port=4
  LL2 : Inport  Port=5
  LL3 : Inport  Port=6
  Control : Subsystem
  Logical Operator : Logic  AllPortsSameDT=off  OutDataTypeStr=boolean
  MasterTankControl : Subsystem
  Memory : Memory
  Memory1 : Memory
  Memory2 : Memory
  TankModel : Subsystem
  LL1 : Outport
  wires:
  TankModel/1(LiquidLevel) -> Memory/1, LL1/1
  Control/1(LiquidIn) -> Logical Operator/1
  Control/2(LiquidOut) -> TankModel/2(LiquidOut)
  Memory/1 -> Control/5(LiquidLevel), MasterTankControl/1(LiquidTank1)
  MR1/1 -> Control/3(ManualReference)
  CT1/1 -> Control/2(StartMaintenance), Control/1(ControlType)
  LL3/1 -> Memory2/1
  Memory2/1 -> MasterTankControl/3(LiquidTank3)
  Memory1/1 -> MasterTankControl/2(LiquidTank2)
  EB1/1 -> Control/4(EmergencyButton)
  MasterTankControl/1(AllowTheTankFilling) -> Logical Operator/2
  Logical Operator/1 -> TankModel/1(LiquidIn)
  LL2/1 -> Memory1/1

== system c00011M_harness/M099/Tank2 ==
  CT2 : Inport
  MR2 : Inport  Port=2
  T2 : Inport  Port=3
  EB2 : Inport  Port=4
  LL1 : Inport  Port=5
  LL3 : Inport  Port=6
  Control : Subsystem
  Logical Operator : Logic  AllPortsSameDT=off  OutDataTypeStr=boolean
  MasterTankControl : Subsystem
  Memory : Memory
  Memory1 : Memory
  Memory2 : Memory
  TankModel : Subsystem
  LL2 : Outport
  wires:
  TankModel/1(LiquidLevel) -> Memory/1, LL2/1
  Control/1(LiquidIn) -> Logical Operator/1
  Control/2(LiquidOut) -> TankModel/2(LiquidOut)
  Memory/1 -> Control/5(LiquidLevel), MasterTankControl/2(LiquidTank2)
  MR2/1 -> Control/3(ManualReference)
  CT2/1 -> Control/2(StartMaintenance), Control/1(ControlType)
  LL3/1 -> Memory2/1
  Memory2/1 -> MasterTankControl/3(LiquidTank3)
  Memory1/1 -> MasterTankControl/1(LiquidTank1)
  EB2/1 -> Control/4(EmergencyButton)
  MasterTankControl/1(AllowTheTankFilling) -> Logical Operator/2
  Logical Operator/1 -> TankModel/1(LiquidIn)
  LL1/1 -> Memory1/1

== system c00011M_harness/M099/Tank3 ==
  CT3 : Inport
  F3 : Inport  Port=2
  E3 : Inport  Port=3
  T3 : Inport  Port=4
  EB3 : Inport  Port=5
  LL1 : Inport  Port=6
  LL2 : Inport  Port=7
  Control : Subsystem
  Logical Operator : Logic  AllPortsSameDT=off  OutDataTypeStr=boolean
  MasterTankControl : Subsystem
  Memory : Memory
  Memory1 : Memory
  Memory2 : Memory
  TankModel : Subsystem
  LL3 : Outport
  wires:
  TankModel/1(LiquidLevel) -> Memory/1, LL3/1
  Control/1(LiquidIn) -> Logical Operator/1
  Control/2(LiquidOut) -> TankModel/2(LiquidOut)
  Memory/1 -> MasterTankControl/3(LiquidTank3), Control/5(LiquidLevel)
  CT3/1 -> Control/1(ControlType)
  F3/1 -> Control/2(Fill)
  E3/1 -> Control/3(Empty)
  LL2/1 -> Memory2/1
  Memory2/1 -> MasterTankControl/2(LiquidTank2)
  Memory1/1 -> MasterTankControl/1(LiquidTank1)
  EB3/1 -> Control/4(EmergencyButton)
  MasterTankControl/1(AllowTheTankFilling) -> Logical Operator/2
  Logical Operator/1 -> TankModel/1(LiquidIn)
  LL1/1 -> Memory1/1

== system c00011M_harness/M100/Tank1 ==
  CT1 : Inport
  MR1 : Inport  Port=2
  T1 : Inport  Port=3
  EB1 : Inport  Port=4
  LL2 : Inport  Port=5
  LL3 : Inport  Port=6
  Control : Subsystem
  Logical Operator : Logic  AllPortsSameDT=off  OutDataTypeStr=boolean
  MasterTankControl : Subsystem
  Memory : Memory
  Memory1 : Memory
  Memory2 : Memory
  TankModel : Subsystem
  LL1 : Outport
  wires:
  TankModel/1(LiquidLevel) -> Memory/1, LL1/1
  Control/1(LiquidIn) -> Logical Operator/1
  Control/2(LiquidOut) -> TankModel/2(LiquidOut)
  Memory/1 -> Control/5(LiquidLevel), MasterTankControl/1(LiquidTank1)
  MR1/1 -> Control/3(ManualReference)
  CT1/1 -> Control/2(StartMaintenance), Control/1(ControlType)
  LL3/1 -> Memory2/1
  Memory2/1 -> MasterTankControl/3(LiquidTank3)
  Memory1/1 -> MasterTankControl/2(LiquidTank2)
  EB1/1 -> Control/4(EmergencyButton)
  MasterTankControl/1(AllowTheTankFilling) -> Logical Operator/2
  Logical Operator/1 -> TankModel/1(LiquidIn)
  LL2/1 -> Memory1/1

== system c00011M_harness/M100/Tank2 ==
  CT2 : Inport
  MR2 : Inport  Port=2
  T2 : Inport  Port=3
  EB2 : Inport  Port=4
  LL1 : Inport  Port=5
  LL3 : Inport  Port=6
  Control : Subsystem
  Logical Operator : Logic  AllPortsSameDT=off  OutDataTypeStr=boolean
  MasterTankControl : Subsystem
  Memory : Memory
  Memory1 : Memory
  Memory2 : Memory
  TankModel : Subsystem
  LL2 : Outport
  wires:
  TankModel/1(LiquidLevel) -> Memory/1, LL2/1
  Control/1(LiquidIn) -> Logical Operator/1
  Control/2(LiquidOut) -> TankModel/2(LiquidOut)
  Memory/1 -> Control/5(LiquidLevel), MasterTankControl/2(LiquidTank2)
  MR2/1 -> Control/3(ManualReference)
  CT2/1 -> Control/2(StartMaintenance), Control/1(ControlType)
  LL3/1 -> Memory2/1
  Memory2/1 -> MasterTankControl/3(LiquidTank3)
  Memory1/1 -> MasterTankControl/1(LiquidTank1)
  EB2/1 -> Control/4(EmergencyButton)
  MasterTankControl/1(AllowTheTankFilling) -> Logical Operator/2
  Logical Operator/1 -> TankModel/1(LiquidIn)
  LL1/1 -> Memory1/1

== system c00011M_harness/M100/Tank3 ==
  CT3 : Inport
  F3 : Inport  Port=2
  E3 : Inport  Port=3
  T3 : Inport  Port=4
  EB3 : Inport  Port=5
  LL1 : Inport  Port=6
  LL2 : Inport  Port=7
  Control : Subsystem
  Logical Operator : Logic  AllPortsSameDT=off  OutDataTypeStr=boolean
  MasterTankControl : Subsystem
  Memory : Memory
  Memory1 : Memory
  Memory2 : Memory
  TankModel : Subsystem
  LL3 : Outport
  wires:
  TankModel/1(LiquidLevel) -> Memory/1, LL3/1
  Control/1(LiquidIn) -> Logical Operator/1
  Control/2(LiquidOut) -> TankModel/2(LiquidOut)
  Memory/1 -> MasterTankControl/3(LiquidTank3), Control/5(LiquidLevel)
  CT3/1 -> Control/1(ControlType)
  F3/1 -> Control/2(Fill)
  E3/1 -> Control/3(Empty)
  LL2/1 -> Memory2/1
  Memory2/1 -> MasterTankControl/2(LiquidTank2)
  Memory1/1 -> MasterTankControl/1(LiquidTank1)
  EB3/1 -> Control/4(EmergencyButton)
  MasterTankControl/1(AllowTheTankFilling) -> Logical Operator/2
  Logical Operator/1 -> TankModel/1(LiquidIn)
  LL1/1 -> Memory1/1

== system c00011M_harness/M101/Tank1 ==
  CT1 : Inport
  MR1 : Inport  Port=2
  T1 : Inport  Port=3
  EB1 : Inport  Port=4
  LL2 : Inport  Port=5
  LL3 : Inport  Port=6
  Control : Subsystem
  Logical Operator : Logic  AllPortsSameDT=off  OutDataTypeStr=boolean
  MasterTankControl : Subsystem
  Memory : Memory
  Memory1 : Memory
  Memory2 : Memory
  TankModel : Subsystem
  LL1 : Outport
  wires:
  TankModel/1(LiquidLevel) -> Memory/1, LL1/1
  Control/1(LiquidIn) -> Logical Operator/1
  Control/2(LiquidOut) -> TankModel/2(LiquidOut)
  Memory/1 -> Control/5(LiquidLevel), MasterTankControl/1(LiquidTank1)
  MR1/1 -> Control/3(ManualReference)
  CT1/1 -> Control/2(StartMaintenance), Control/1(ControlType)
  LL3/1 -> Memory2/1
  Memory2/1 -> MasterTankControl/3(LiquidTank3)
  Memory1/1 -> MasterTankControl/2(LiquidTank2)
  EB1/1 -> Control/4(EmergencyButton)
  MasterTankControl/1(AllowTheTankFilling) -> Logical Operator/2
  Logical Operator/1 -> TankModel/1(LiquidIn)
  LL2/1 -> Memory1/1

== system c00011M_harness/M101/Tank2 ==
  CT2 : Inport
  MR2 : Inport  Port=2
  T2 : Inport  Port=3
  EB2 : Inport  Port=4
  LL1 : Inport  Port=5
  LL3 : Inport  Port=6
  Control : Subsystem
  Logical Operator : Logic  AllPortsSameDT=off  OutDataTypeStr=boolean
  MasterTankControl : Subsystem
  Memory : Memory
  Memory1 : Memory
  Memory2 : Memory
  TankModel : Subsystem
  LL2 : Outport
  wires:
  TankModel/1(LiquidLevel) -> Memory/1, LL2/1
  Control/1(LiquidIn) -> Logical Operator/1
  Control/2(LiquidOut) -> TankModel/2(LiquidOut)
  Memory/1 -> Control/5(LiquidLevel), MasterTankControl/2(LiquidTank2)
  MR2/1 -> Control/3(ManualReference)
  CT2/1 -> Control/2(StartMaintenance), Control/1(ControlType)
  LL3/1 -> Memory2/1
  Memory2/1 -> MasterTankControl/3(LiquidTank3)
  Memory1/1 -> MasterTankControl/1(LiquidTank1)
  EB2/1 -> Control/4(EmergencyButton)
  MasterTankControl/1(AllowTheTankFilling) -> Logical Operator/2
  Logical Operator/1 -> TankModel/1(LiquidIn)
  LL1/1 -> Memory1/1

== system c00011M_harness/M101/Tank3 ==
  CT3 : Inport
  F3 : Inport  Port=2
  E3 : Inport  Port=3
  T3 : Inport  Port=4
  EB3 : Inport  Port=5
  LL1 : Inport  Port=6
  LL2 : Inport  Port=7
  Control : Subsystem
  Logical Operator : Logic  AllPortsSameDT=off  OutDataTypeStr=boolean
  MasterTankControl : Subsystem
  Memory : Memory
  Memory1 : Memory
  Memory2 : Memory
  TankModel : Subsystem
  LL3 : Outport
  wires:
  TankModel/1(LiquidLevel) -> Memory/1, LL3/1
  Control/1(LiquidIn) -> Logical Operator/1
  Control/2(LiquidOut) -> TankModel/2(LiquidOut)
  Memory/1 -> MasterTankControl/3(LiquidTank3), Control/5(LiquidLevel)
  CT3/1 -> Control/1(ControlType)
  F3/1 -> Control/2(Fill)
  E3/1 -> Control/3(Empty)
  LL2/1 -> Memory2/1
  Memory2/1 -> MasterTankControl/2(LiquidTank2)
  Memory1/1 -> MasterTankControl/1(LiquidTank1)
  EB3/1 -> Control/4(EmergencyButton)
  MasterTankControl/1(AllowTheTankFilling) -> Logical Operator/2
  Logical Operator/1 -> TankModel/1(LiquidIn)
  LL1/1 -> Memory1/1

== system c00011M_harness/M102/Tank1 ==
  CT1 : Inport
  MR1 : Inport  Port=2
  T1 : Inport  Port=3
  EB1 : Inport  Port=4
  LL2 : Inport  Port=5
  LL3 : Inport  Port=6
  Control : Subsystem
  Logical Operator : Logic  AllPortsSameDT=off  OutDataTypeStr=boolean
  MasterTankControl : Subsystem
  Memory : Memory
  Memory1 : Memory
  Memory2 : Memory
  TankModel : Subsystem
  LL1 : Outport
  wires:
  TankModel/1(LiquidLevel) -> Memory/1, LL1/1
  Control/1(LiquidIn) -> Logical Operator/1
  Control/2(LiquidOut) -> TankModel/2(LiquidOut)
  Memory/1 -> Control/5(LiquidLevel), MasterTankControl/1(LiquidTank1)
  MR1/1 -> Control/3(ManualReference)
  CT1/1 -> Control/2(StartMaintenance), Control/1(ControlType)
  LL3/1 -> Memory2/1
  Memory2/1 -> MasterTankControl/3(LiquidTank3)
  Memory1/1 -> MasterTankControl/2(LiquidTank2)
  EB1/1 -> Control/4(EmergencyButton)
  MasterTankControl/1(AllowTheTankFilling) -> Logical Operator/2
  Logical Operator/1 -> TankModel/1(LiquidIn)
  LL2/1 -> Memory1/1

== system c00011M_harness/M102/Tank2 ==
  CT2 : Inport
  MR2 : Inport  Port=2
  T2 : Inport  Port=3
  EB2 : Inport  Port=4
  LL1 : Inport  Port=5
  LL3 : Inport  Port=6
  Control : Subsystem
  Logical Operator : Logic  AllPortsSameDT=off  OutDataTypeStr=boolean
  MasterTankControl : Subsystem
  Memory : Memory
  Memory1 : Memory
  Memory2 : Memory
  TankModel : Subsystem
  LL2 : Outport
  wires:
  TankModel/1(LiquidLevel) -> Memory/1, LL2/1
  Control/1(LiquidIn) -> Logical Operator/1
  Control/2(LiquidOut) -> TankModel/2(LiquidOut)
  Memory/1 -> Control/5(LiquidLevel), MasterTankControl/2(LiquidTank2)
  MR2/1 -> Control/3(ManualReference)
  CT2/1 -> Control/2(StartMaintenance), Control/1(ControlType)
  LL3/1 -> Memory2/1
  Memory2/1 -> MasterTankControl/3(LiquidTank3)
  Memory1/1 -> MasterTankControl/1(LiquidTank1)
  EB2/1 -> Control/4(EmergencyButton)
  MasterTankControl/1(AllowTheTankFilling) -> Logical Operator/2
  Logical Operator/1 -> TankModel/1(LiquidIn)
  LL1/1 -> Memory1/1

== system c00011M_harness/M102/Tank3 ==
  CT3 : Inport
  F3 : Inport  Port=2
  E3 : Inport  Port=3
  T3 : Inport  Port=4
  EB3 : Inport  Port=5
  LL1 : Inport  Port=6
  LL2 : Inport  Port=7
  Control : Subsystem
  Logical Operator : Logic  AllPortsSameDT=off  OutDataTypeStr=boolean
  MasterTankControl : Subsystem
  Memory : Memory
  Memory1 : Memory
  Memory2 : Memory
  TankModel : Subsystem
  LL3 : Outport
  wires:
  TankModel/1(LiquidLevel) -> Memory/1, LL3/1
  Control/1(LiquidIn) -> Logical Operator/1
  Control/2(LiquidOut) -> TankModel/2(LiquidOut)
  Memory/1 -> MasterTankControl/3(LiquidTank3), Control/5(LiquidLevel)
  CT3/1 -> Control/1(ControlType)
  F3/1 -> Control/2(Fill)
  E3/1 -> Control/3(Empty)
  LL2/1 -> Memory2/1
  Memory2/1 -> MasterTankControl/2(LiquidTank2)
  Memory1/1 -> MasterTankControl/1(LiquidTank1)
  EB3/1 -> Control/4(EmergencyButton)
  MasterTankControl/1(AllowTheTankFilling) -> Logical Operator/2
  Logical Operator/1 -> TankModel/1(LiquidIn)
  LL1/1 -> Memory1/1

== system c00011M_harness/M103/Tank1 ==
  CT1 : Inport
  MR1 : Inport  Port=2
  T1 : Inport  Port=3
  EB1 : Inport  Port=4
  LL2 : Inport  Port=5
  LL3 : Inport  Port=6
  Control : Subsystem
  Logical Operator : Logic  AllPortsSameDT=off  OutDataTypeStr=boolean
  MasterTankControl : Subsystem
  Memory : Memory
  Memory1 : Memory
  Memory2 : Memory
  TankModel : Subsystem
  LL1 : Outport
  wires:
  TankModel/1(LiquidLevel) -> Memory/1, LL1/1
  Control/1(LiquidIn) -> Logical Operator/1
  Control/2(LiquidOut) -> TankModel/2(LiquidOut)
  Memory/1 -> Control/5(LiquidLevel), MasterTankControl/1(LiquidTank1)
  MR1/1 -> Control/3(ManualReference)
  CT1/1 -> Control/2(StartMaintenance), Control/1(ControlType)
  LL3/1 -> Memory2/1
  Memory2/1 -> MasterTankControl/3(LiquidTank3)
  Memory1/1 -> MasterTankControl/2(LiquidTank2)
  EB1/1 -> Control/4(EmergencyButton)
  MasterTankControl/1(AllowTheTankFilling) -> Logical Operator/2
  Logical Operator/1 -> TankModel/1(LiquidIn)
  LL2/1 -> Memory1/1

== system c00011M_harness/M103/Tank2 ==
  CT2 : Inport
  MR2 : Inport  Port=2
  T2 : Inport  Port=3
  EB2 : Inport  Port=4
  LL1 : Inport  Port=5
  LL3 : Inport  Port=6
  Control : Subsystem
  Logical Operator : Logic  AllPortsSameDT=off  OutDataTypeStr=boolean
  MasterTankControl : Subsystem
  Memory : Memory
  Memory1 : Memory
  Memory2 : Memory
  TankModel : Subsystem
  LL2 : Outport
  wires:
  TankModel/1(LiquidLevel) -> Memory/1, LL2/1
  Control/1(LiquidIn) -> Logical Operator/1
  Control/2(LiquidOut) -> TankModel/2(LiquidOut)
  Memory/1 -> Control/5(LiquidLevel), MasterTankControl/2(LiquidTank2)
  MR2/1 -> Control/3(ManualReference)
  CT2/1 -> Control/2(StartMaintenance), Control/1(ControlType)
  LL3/1 -> Memory2/1
  Memory2/1 -> MasterTankControl/3(LiquidTank3)
  Memory1/1 -> MasterTankControl/1(LiquidTank1)
  EB2/1 -> Control/4(EmergencyButton)
  MasterTankControl/1(AllowTheTankFilling) -> Logical Operator/2
  Logical Operator/1 -> TankModel/1(LiquidIn)
  LL1/1 -> Memory1/1

== system c00011M_harness/M103/Tank3 ==
  CT3 : Inport
  F3 : Inport  Port=2
  E3 : Inport  Port=3
  T3 : Inport  Port=4
  EB3 : Inport  Port=5
  LL1 : Inport  Port=6
  LL2 : Inport  Port=7
  Control : Subsystem
  Logical Operator : Logic  AllPortsSameDT=off  OutDataTypeStr=boolean
  MasterTankControl : Subsystem
  Memory : Memory
  Memory1 : Memory
  Memory2 : Memory
  TankModel : Subsystem
  LL3 : Outport
  wires:
  TankModel/1(LiquidLevel) -> Memory/1, LL3/1
  Control/1(LiquidIn) -> Logical Operator/1
  Control/2(LiquidOut) -> TankModel/2(LiquidOut)
  Memory/1 -> MasterTankControl/3(LiquidTank3), Control/5(LiquidLevel)
  CT3/1 -> Control/1(ControlType)
  F3/1 -> Control/2(Fill)
  E3/1 -> Control/3(Empty)
  LL2/1 -> Memory2/1
  Memory2/1 -> MasterTankControl/2(LiquidTank2)
  Memory1/1 -> MasterTankControl/1(LiquidTank1)
  EB3/1 -> Control/4(EmergencyButton)
  MasterTankControl/1(AllowTheTankFilling) -> Logical Operator/2
  Logical Operator/1 -> TankModel/1(LiquidIn)
  LL1/1 -> Memory1/1

== system c00011M_harness/M104/Tank1 ==
  CT1 : Inport
  MR1 : Inport  Port=2
  T1 : Inport  Port=3
  EB1 : Inport  Port=4
  LL2 : Inport  Port=5
  LL3 : Inport  Port=6
  Control : Subsystem
  Logical Operator : Logic  AllPortsSameDT=off  OutDataTypeStr=boolean
  MasterTankControl : Subsystem
  Memory : Memory
  Memory1 : Memory
  Memory2 : Memory
  TankModel : Subsystem
  LL1 : Outport
  wires:
  TankModel/1(LiquidLevel) -> Memory/1, LL1/1
  Control/1(LiquidIn) -> Logical Operator/1
  Control/2(LiquidOut) -> TankModel/2(LiquidOut)
  Memory/1 -> Control/5(LiquidLevel), MasterTankControl/1(LiquidTank1)
  MR1/1 -> Control/3(ManualReference)
  CT1/1 -> Control/2(StartMaintenance), Control/1(ControlType)
  LL3/1 -> Memory2/1
  Memory2/1 -> MasterTankControl/3(LiquidTank3)
  Memory1/1 -> MasterTankControl/2(LiquidTank2)
  EB1/1 -> Control/4(EmergencyButton)
  MasterTankControl/1(AllowTheTankFilling) -> Logical Operator/2
  Logical Operator/1 -> TankModel/1(LiquidIn)
  LL2/1 -> Memory1/1

== system c00011M_harness/M104/Tank2 ==
  CT2 : Inport
  MR2 : Inport  Port=2
  T2 : Inport  Port=3
  EB2 : Inport  Port=4
  LL1 : Inport  Port=5
  LL3 : Inport  Port=6
  Control : Subsystem
  Logical Operator : Logic  AllPortsSameDT=off  OutDataTypeStr=boolean
  MasterTankControl : Subsystem
  Memory : Memory
  Memory1 : Memory
  Memory2 : Memory
  TankModel : Subsystem
  LL2 : Outport
  wires:
  TankModel/1(LiquidLevel) -> Memory/1, LL2/1
  Control/1(LiquidIn) -> Logical Operator/1
  Control/2(LiquidOut) -> TankModel/2(LiquidOut)
  Memory/1 -> Control/5(LiquidLevel), MasterTankControl/2(LiquidTank2)
  MR2/1 -> Control/3(ManualReference)
  CT2/1 -> Control/2(StartMaintenance), Control/1(ControlType)
  LL3/1 -> Memory2/1
  Memory2/1 -> MasterTankControl/3(LiquidTank3)
  Memory1/1 -> MasterTankControl/1(LiquidTank1)
  EB2/1 -> Control/4(EmergencyButton)
  MasterTankControl/1(AllowTheTankFilling) -> Logical Operator/2
  Logical Operator/1 -> TankModel/1(LiquidIn)
  LL1/1 -> Memory1/1
